simulink model "VTOL_sim_broke"  (R2015a)
settings: Solver=ode45  StartTime=0.0  StopTime=200  RelTol=1e-3
InitFcn:
  | param
undefined symbols (not defined in the file or in its folder): drawVTOL, P, Planar_VTOL_SSctrl
settings Model: Creator=beard  LastModifiedBy=ecestudent
settings DataIOCC: SignalLoggingSaveFormat=ModelDataLogs
settings OptimizationCC: ExpressionDepthLimit=2147483647  InitFltsAndDblsToZero=on
settings DebuggingCC: UnderspecifiedInitializationDetection=Classic  MergeDetectMultiDrivingBlocksExec=none  SolverPrmCheckMsg=warning  FcnCallInpInsideContextMsg=UseLocalSettings  StateNameClashWarn=warning
settings GRTTargetCC: CombineOutputUpdateFcns=off  GRTInterface=on

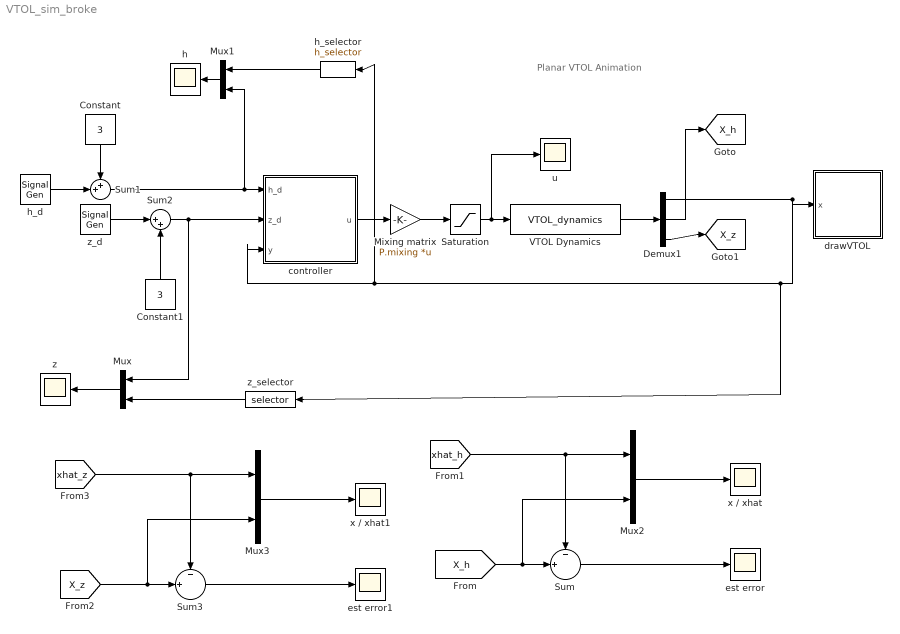
== system VTOL_sim_broke ==
  note: Planar VTOL Animation
  Constant : Constant  Value=3
  Constant1 : Constant  Value=3
  Demux1 : Demux  Outputs=[3 2 4]
  Mixing matrix : Gain  Gain=P.mixing  Multiplication=Matrix(K*u)
  Mux{,1..3} (4 alike) : Mux  Inputs=2
  Saturation : Saturate  UpperLimit=P.fmax  LowerLimit=0
  Sum : Sum  Inputs=-|+||
  Sum1 : Sum  Inputs=++|
  Sum2 : Sum  Inputs=|++
  Sum3 : Sum  Inputs=-|+||
  VTOL Dynamics : S-Function  FunctionName=VTOL_dynamics  Parameters=AP
  controller : Subsystem
  drawVTOL : Subsystem
      mask Display: image(imread('tv.jpg'))
  est error : Scope
      settings: TimeRange=200  YMin=-0.5  YMax=0.3  SaveName=ScopeData6
  est error1 : Scope
      settings: TimeRange=200  YMin=-0.5  YMax=0.3  SaveName=ScopeData8
  h : Scope
      settings: YMin=0  YMax=65
  h_d : SignalGenerator  WaveForm=square  Amplitude=2.5  Frequency=.02
  h_selector : MATLABFcn  MATLABFcn=h_selector  OutputDimensions=1
  u : Scope
      settings: TimeRange=200  YMin=6  YMax=10  SaveName=ScopeData2
  x / xhat : Scope
      settings: YMin=-0.2  YMax=0.5  SaveName=ScopeData7
  x / xhat1 : Scope
      settings: YMin=-0.2  YMax=0.5  SaveName=ScopeData9
  z : Scope
      settings: YMin=0  YMax=5.75
  z_d : SignalGenerator  WaveForm=square  Amplitude=2.5  Frequency=.008
  z_selector : MATLABFcn  MATLABFcn=selector  OutputDimensions=1
  tag scope: X_h=global, X_z=global
  wires:
  Constant/1 -> Sum1/1
  h_d/1 -> Sum1/2
  Sum2/1 -> Mux/1, controller/2(z_d)
  z_d/1 -> Sum2/1
  Constant1/1 -> Sum2/2
  Saturation/1 -> u/1, VTOL Dynamics/1
  Mixing matrix/1 -> Saturation/1
  controller/1(u) -> Mixing matrix/1
  Sum1/1 -> Mux1/2, controller/1(h_d)
  Mux/1 -> z/1
  z_selector/1 -> Mux/2
  Mux1/1 -> h/1
  h_selector/1 -> Mux1/1
  VTOL Dynamics/1 -> Demux1/1
  Demux1/1 -> z_selector/1, h_selector/1, controller/3(y), drawVTOL/1(x)
  Demux1/2 -> [X_h]
  [X_h] -> Mux2/2, Sum/2
  [xhat_h] -> Sum/1, Mux2/1
  Mux2/1 -> x / xhat/1
  Sum/1 -> est error/1
  [X_z] -> Mux3/2, Sum3/2
  [xhat_z] -> Sum3/1, Mux3/1
  Mux3/1 -> x / xhat1/1
  Sum3/1 -> est error1/1
  Demux1/3 -> [X_z]

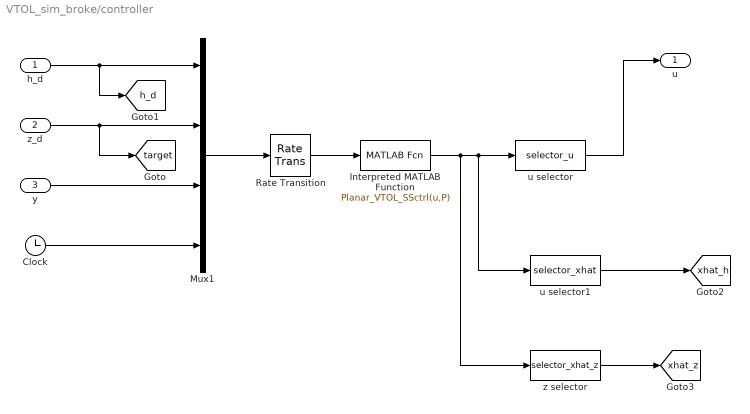
== system VTOL_sim_broke/controller ==
  h_d : Inport
  z_d : Inport  Port=2
  y : Inport  Port=3
  Clock : Clock
  Interpreted MATLAB Function : MATLABFcn  MATLABFcn=Planar_VTOL_SSctrl(u,P)  OutputDimensions=8
  Mux1 : Mux
  Rate Transition : RateTransition  OutPortSampleTime=P.Ts
  u selector : MATLABFcn  MATLABFcn=selector_u  OutputDimensions=2
  u selector1 : MATLABFcn  MATLABFcn=selector_xhat  OutputDimensions=1
  z selector : MATLABFcn  MATLABFcn=selector_xhat_z  OutputDimensions=1
  u : Outport
  tag scope: h_d=global, target=global, xhat_h=global, xhat_z=global
  wires:
  Mux1/1 -> Rate Transition/1
  h_d/1 -> [h_d], Mux1/1
  Clock/1 -> Mux1/4
  Rate Transition/1 -> Interpreted MATLAB Function/1
  y/1 -> Mux1/3
  z_d/1 -> [target], Mux1/2
  Interpreted MATLAB Function/1 -> z selector/1, u selector1/1, u selector/1
  u selector/1 -> u/1
  u selector1/1 -> [xhat_h]
  z selector/1 -> [xhat_z]

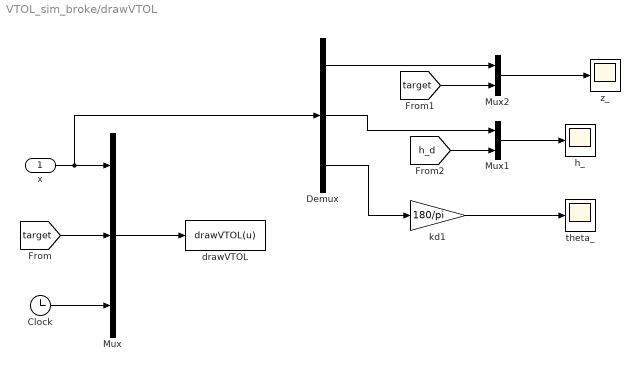
== system VTOL_sim_broke/drawVTOL ==
  x : Inport
  Clock : Clock
  Demux : Demux  Outputs=3
  Mux : Mux  Inputs=3
  Mux1 : Mux  Inputs=2
  Mux2 : Mux  Inputs=2
  drawVTOL : MATLABFcn  MATLABFcn=drawVTOL(u)  OutputDimensions=0  SampleTime=0.1
  h_ : Scope
      settings: TimeRange=200  YMin=0  YMax=6  SaveName=ScopeData3
  kd1 : Gain  Gain=180/pi
  theta_ : Scope
      settings: TimeRange=200  YMin=-60  YMax=60  SaveName=ScopeData5
  z_ : Scope
      settings: TimeRange=200  YMin=0  YMax=6  SaveName=ScopeData4
  wires:
  Mux/1 -> drawVTOL/1
  x/1 -> Demux/1, Mux/1
  Clock/1 -> Mux/3
  [target] -> Mux/2
  Mux1/1 -> h_/1
  Mux2/1 -> z_/1
  kd1/1 -> theta_/1
  Demux/3 -> kd1/1
  Demux/1 -> Mux2/1
  [target] -> Mux2/2
  Demux/2 -> Mux1/1
  [h_d] -> Mux1/2
